simulink model "test_model"  (Simulink 8.3)
settings: Solver=VariableStepDiscrete  StartTime=0.0  StopTime=1999  RelTol=1e-3
values from neighbouring files (symbols this model uses):
  den = [1 -1.47368785983 1.00754704055 -0.135335283237]    [plantData.mat]    (also in test_case1.m = cell2mat(sysd.den))
  num = [0 0.657515824638 0.0420150742993 0.496040793515]    [plantData.mat]    (also in test_case1.m = cell2mat(sysd.num))
  Ts = 1    [compareTestcase.m]    (also in plantData.mat; test_case1.m = sysd.Ts)
settings Model: Creator=Ravan  LastModifiedBy=Ravan
settings DataIOCC: SignalLoggingSaveFormat=Dataset
settings DebuggingCC: UnderspecifiedInitializationDetection=Simplified  SolverPrmCheckMsg=none  StateNameClashWarn=none
settings GRTTargetCC: CombineOutputUpdateFcns=on  GRTInterface=off

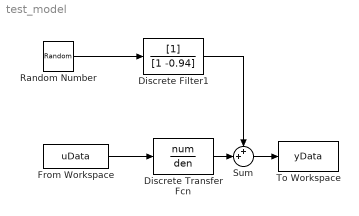
== system test_model ==
  Discrete Transfer Fcn : DiscreteTransferFcn  Numerator=num  Denominator=den  SampleTime=Ts
  Discrete Filter1 : DiscreteFilter  Denominator=[1 -0.94]  SampleTime=Ts
  From Workspace : FromWorkspace  VariableName=uData  SampleTime=Ts
  Random Number : RandomNumber  Variance=0.1  SampleTime=1
  Sum : Sum  Inputs=++|
  To Workspace : ToWorkspace  VariableName=yData  SaveFormat=Timeseries  SampleTime=Ts
  wires:
  From Workspace/1 -> Discrete Transfer Fcn/1
  Random Number/1 -> Discrete Filter1/1
  Discrete Filter1/1 -> Sum/1
  Discrete Transfer Fcn/1 -> Sum/2
  Sum/1 -> To Workspace/1
